simulink model "modelo_dinamico_LAB"  (R2024b)
settings: Solver=FixedStepAuto  StartTime=0.0  StopTime=end_time-Ts  FixedStep=Ts  RelTol=1e-3
undefined symbols (not defined in the file): g, M, tau_phi_max, tau_phi_min, tau_psi_max, tau_psi_min, tau_theta_max, tau_theta_min, Ts, u_max, u_min, x11_0, x1_0, x3_0, x5_0, x7_0, x9_0
libraries: slident x1
settings Model: Creator=pdelr  LastModifiedBy=pdelr
settings DebuggingCC: UnconnectedInputMsg=warning  UnconnectedOutputMsg=warning  UnconnectedLineMsg=warning
settings ModelReferenceCC: EnableRefExpFcnMdlSchedulingChecks=on
settings RTWCC: GPUComputeCapability=3.5  DLArmComputeVersion=19.05

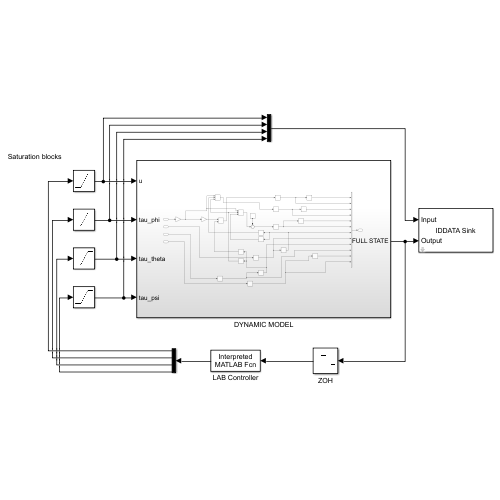
[thumbnail: Simulink's stored preview of the top-level diagram]
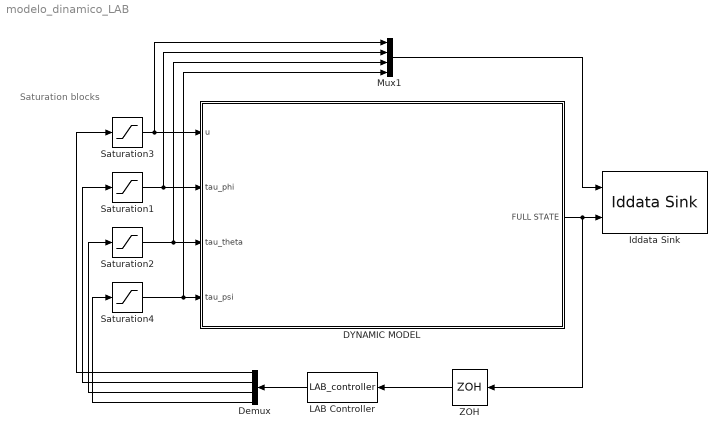
== system modelo_dinamico_LAB ==
  note: Saturation blocks
  DYNAMIC MODEL : Subsystem
  Demux : Demux
  Iddata Sink : slident/Iddata Sink  datasetname=data  Ts=Ts  isu=on  isy=on
  LAB Controller : MATLABFcn  MATLABFcn=LAB_controller  OutputDimensions=4
  Mux1 : Mux
  Saturation1 : Saturate  UpperLimit=tau_phi_max  LowerLimit=tau_phi_min
  Saturation2 : Saturate  UpperLimit=tau_theta_max  LowerLimit=tau_theta_min
  Saturation3 : Saturate  UpperLimit=u_max  LowerLimit=u_min
  Saturation4 : Saturate  UpperLimit=tau_psi_max  LowerLimit=tau_psi_min
  ZOH : ZeroOrderHold  SampleTime=Ts
  wires:
  Demux/1 -> Saturation3/1
  Demux/2 -> Saturation1/1
  Demux/4 -> Saturation4/1
  Demux/3 -> Saturation2/1
  Mux1/1 -> Iddata Sink/1
  Saturation3/1 -> DYNAMIC MODEL/1(u), Mux1/1
  Saturation1/1 -> DYNAMIC MODEL/2(tau_phi), Mux1/2
  Saturation2/1 -> DYNAMIC MODEL/3(tau_theta), Mux1/3
  Saturation4/1 -> DYNAMIC MODEL/4(tau_psi), Mux1/4
  LAB Controller/1 -> Demux/1
  ZOH/1 -> LAB Controller/1
  DYNAMIC MODEL/1(FULL STATE) -> ZOH/1, Iddata Sink/2

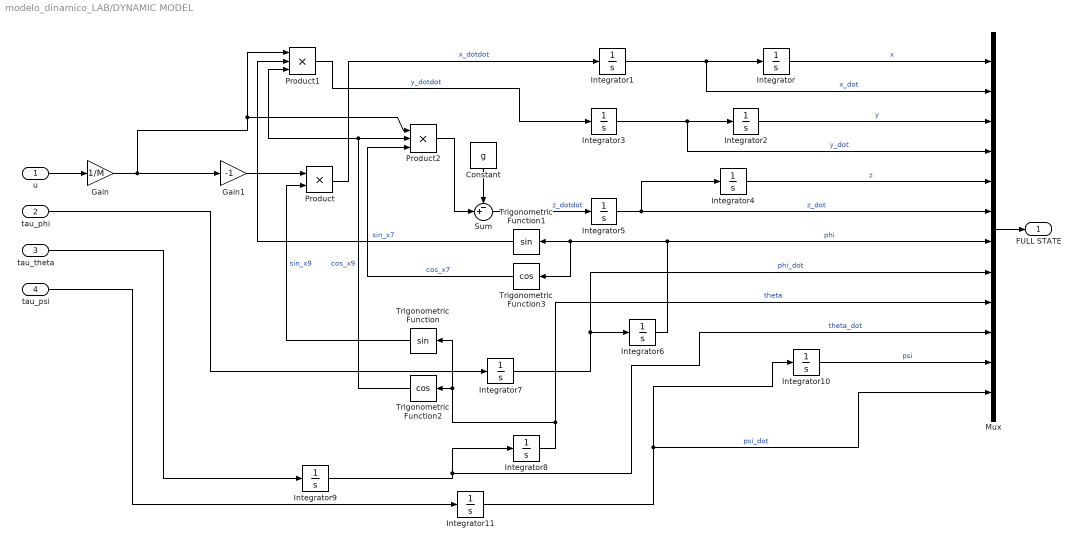
== system modelo_dinamico_LAB/DYNAMIC MODEL ==
  u : Inport
  tau_phi : Inport  Port=2
  tau_theta : Inport  Port=3
  tau_psi : Inport  Port=4
  Constant : Constant  Value=g
  Gain : Gain  Gain=1/M
  Gain1 : Gain  Gain=-1
  Integrator : Integrator  InitialCondition=x1_0
  Integrator{1,3,5,7,9,11} (6 alike) : Integrator
  Integrator10 : Integrator  InitialCondition=x11_0
  Integrator2 : Integrator  InitialCondition=x3_0
  Integrator4 : Integrator  InitialCondition=x5_0
  Integrator6 : Integrator  InitialCondition=x7_0
  Integrator8 : Integrator  InitialCondition=x9_0
  Mux : Mux  Inputs=12
  Product : Product
  Product1 : Product  Inputs=3
  Product2 : Product  Inputs=3
  Sum : Sum  Inputs=-+|
  Trigonometric Function : Trigonometry
  Trigonometric Function1 : Trigonometry
  Trigonometric Function2 : Trigonometry  Operator=cos
  Trigonometric Function3 : Trigonometry  Operator=cos
  FULL STATE : Outport
  wires:
  Integrator5/1 -> Integrator4/1, Mux/6  "z_dot"
  Integrator8/1 -> Mux/9, Trigonometric Function2/1, Trigonometric Function/1  "theta"
  Integrator3/1 -> Mux/4, Integrator2/1  "y_dot"
  Integrator7/1 -> Integrator6/1, Mux/8  "phi_dot"
  Trigonometric Function3/1 -> Product2/3  "cos_x7"
  Integrator2/1 -> Mux/3  "y"
  Integrator6/1 -> Trigonometric Function3/1, Trigonometric Function1/1, Mux/7  "phi"
  Integrator9/1 -> Mux/10, Integrator8/1  "theta_dot"
  Product1/1 -> Integrator3/1  "y_dotdot"
  Product/1 -> Integrator1/1  "x_dotdot"
  Trigonometric Function/1 -> Product/2  "sin_x9"
  Integrator/1 -> Mux/1  "x"
  Trigonometric Function1/1 -> Product1/2  "sin_x7"
  Integrator4/1 -> Mux/5  "z"
  Trigonometric Function2/1 -> Product2/2, Product1/3  "cos_x9"
  Integrator11/1 -> Integrator10/1, Mux/12  "psi_dot"
  Integrator1/1 -> Mux/2, Integrator/1  "x_dot"
  Gain/1 -> Gain1/1, Product1/1, Product2/1
  Integrator10/1 -> Mux/11  "psi"
  Gain1/1 -> Product/1
  Sum/1 -> Integrator5/1  "z_dotdot"
  Product2/1 -> Sum/2
  Constant/1 -> Sum/1
  Mux/1 -> FULL STATE/1
  tau_phi/1 -> Integrator7/1
  tau_theta/1 -> Integrator9/1
  tau_psi/1 -> Integrator11/1
  u/1 -> Gain/1
